simulink model "AV_7_zadaca2_baranje1"  (R2018a)
settings: Solver=VariableStepAuto  StartTime=0.0  StopTime=50  RelTol=1e-3
libraries: simulink_extras x1
settings Model: Creator=DD  LastModifiedBy=DD

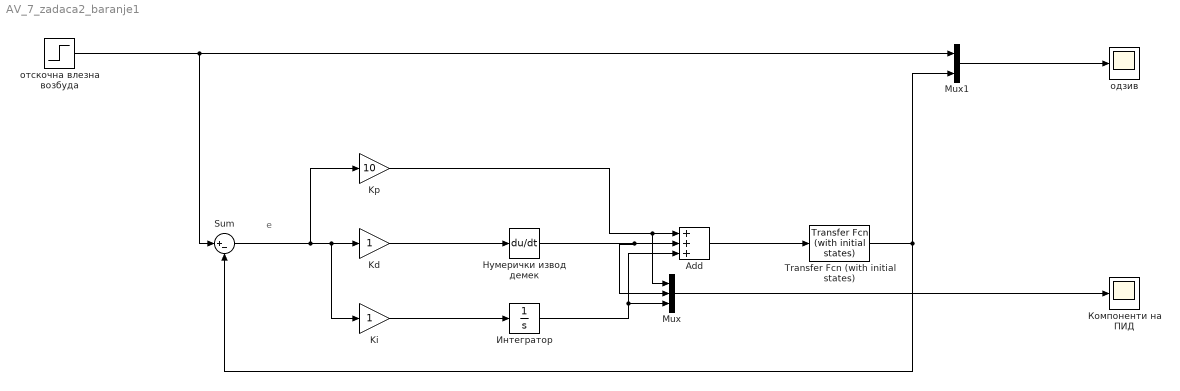
== system AV_7_zadaca2_baranje1 ==
  note: е
  Add : Sum  Inputs=+++
  Kd : Gain
  "Ki " : Gain
  Kp : Gain  Gain=10
  Mux : Mux  Inputs=3
  Mux1 : Mux  Inputs=2
  Sum : Sum  Inputs=|+-
  Transfer Fcn (with initial states) : simulink_extras/Additional Linear/Transfer Fcn (with initial states)  N=[1]  D="[1  10 20]"  X0=0.1
  "Интегратор " : Integrator
  Компоненти на ПИД : Scope
  "Нумерички извод демек " : Derivative
  одзив : Scope
  "отскочна влезна возбуда " : Step  SampleTime=0
  wires:
  Kd/1 -> "Нумерички извод демек "/1
  "Ki "/1 -> "Интегратор "/1
  "Нумерички извод демек "/1 -> Mux/2, Add/2
  Kp/1 -> Mux/1, Add/1
  "Интегратор "/1 -> Mux/3, Add/3
  Add/1 -> Transfer Fcn (with initial states)/1
  Transfer Fcn (with initial states)/1 -> Sum/2, Mux1/2
  "отскочна влезна возбуда "/1 -> Sum/1, Mux1/1
  Mux/1 -> Компоненти на ПИД/1
  Mux1/1 -> одзив/1
  Sum/1 -> Kp/1, "Ki "/1, Kd/1
